simulink model "week1prob9"  (R2020b)
settings: Solver=VariableStepAuto  StartTime=0.0  StopTime=10.0  RelTol=1e-3
model workspace (MAT data in the model file):
  J = Simulink.Parameter
  J.Value = 0.01
  J.DataType = 'auto'
  J.Dimensions = [1 1]
  K = Simulink.Parameter
  K.Value = 0.01
  K.DataType = 'auto'
  K.Dimensions = [1 1]
  L = Simulink.Parameter
  L.Value = 0.5
  L.DataType = 'auto'
  L.Dimensions = [1 1]
  R = Simulink.Parameter
  R.Value = 1
  R.DataType = 'auto'
  R.Dimensions = [1 1]
  b = Simulink.Parameter
  b.Value = 0.1
  b.DataType = 'auto'
  b.Dimensions = [1 1]
settings Model: Creator=lalit  LastModifiedBy=lalit

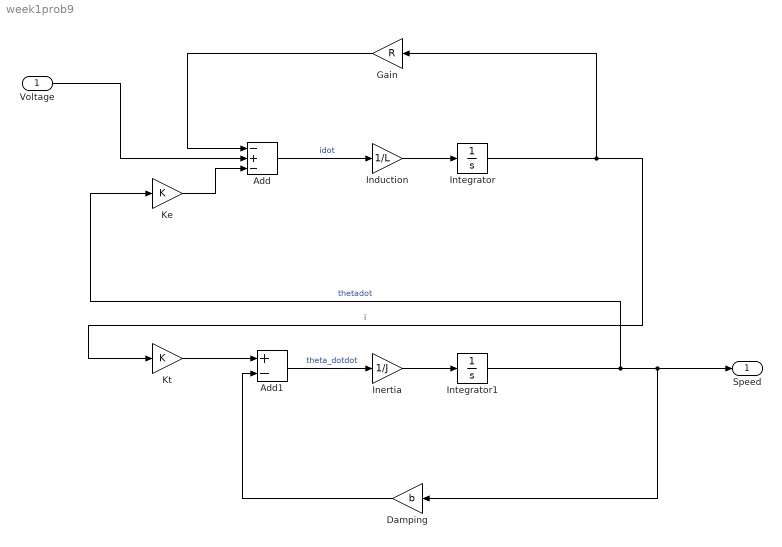
== system week1prob9 ==
  Voltage : Inport
  Add : Sum  Inputs=-+-
  Add1 : Sum  Inputs=+-
  Damping : Gain  Gain=b
  Gain : Gain  Gain=R
  Induction : Gain  Gain=1/L
  Inertia : Gain  Gain=1/J
  Integrator : Integrator
  Integrator1 : Integrator
  Ke : Gain  Gain=K
  Kt : Gain  Gain=K
  Speed : Outport
  wires:
  Integrator/1 -> Gain/1, Kt/1  "i"
  Add/1 -> Induction/1  "idot"
  Integrator1/1 -> Ke/1, Speed/1, Damping/1  "thetadot"
  Add1/1 -> Inertia/1  "theta_dotdot"
  Induction/1 -> Integrator/1
  Inertia/1 -> Integrator1/1
  Kt/1 -> Add1/1
  Damping/1 -> Add1/2
  Gain/1 -> Add/1
  Ke/1 -> Add/3
  Voltage/1 -> Add/2
